simulink model "lab4_G_coeff_model_for_estimation_2019b"  (R2019b)
settings: Solver=FixedStepAuto  StartTime=0.0  StopTime=60  FixedStep=0.01  RelTol=1e-3
model workspace (MAT data in the model file):
  lab4_G_coeff_model_for_estimation_spesession : sldodialogs.data.SessionData (value not decoded)
undefined symbols (not defined in the file or in its folder): G, p
settings Model: OrderedModelArguments=off  Creator=STUDENT  LastModifiedBy=dawid

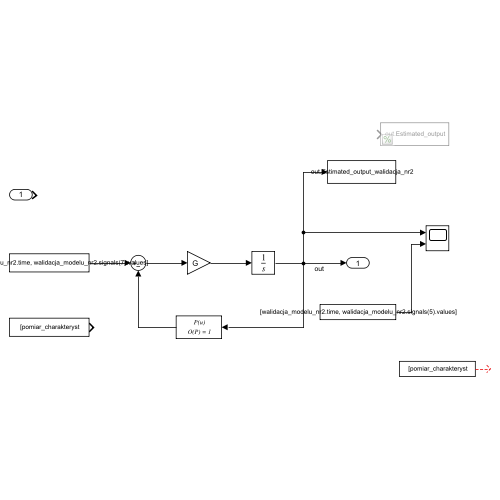
[thumbnail: Simulink's stored preview of the top-level diagram]
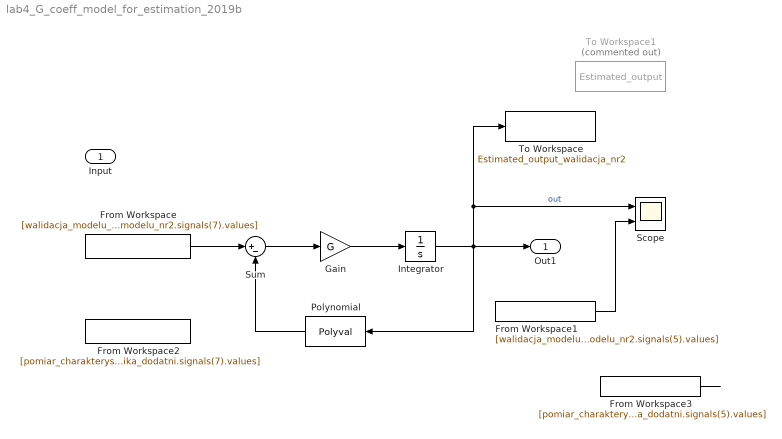
== system lab4_G_coeff_model_for_estimation_2019b ==
  Input : Inport
  From Workspace : FromWorkspace  VariableName=[walidacja_modelu_nr2.time, walidacja_modelu_nr2.signals(7).values]
  From Workspace1 : FromWorkspace  VariableName=[walidacja_modelu_nr2.time, walidacja_modelu_nr2.signals(5).values]
  From Workspace2 : FromWorkspace  VariableName=[pomiar_charakterystyki_silnika_dodatni.time, pomiar_charakterystyki_silnika_dodatni.signals(7).values]
  From Workspace3 : FromWorkspace  VariableName=[pomiar_charakterystyki_silnika_dodatni.time, pomiar_charakterystyki_silnika_dodatni.signals(5).values]
  Gain : Gain  Gain=G
  Integrator : Integrator
  Polynomial : Polyval  Coefs=p
  Scope : Scope  NumInputPorts=2
  Sum : Sum  Inputs=|+-
  To Workspace : ToWorkspace  VariableName=Estimated_output_walidacja_nr2  SaveFormat=Timeseries  SampleTime=-1
  To Workspace1 : ToWorkspace  Commented=on  VariableName=Estimated_output  SaveFormat=Timeseries  SampleTime=-1
  Out1 : Outport
  wires:
  Sum/1 -> Gain/1
  Gain/1 -> Integrator/1
  Integrator/1 -> To Workspace/1, Scope/1, Polynomial/1, Out1/1  "out"
  Polynomial/1 -> Sum/2
  From Workspace1/1 -> Scope/2
  From Workspace/1 -> Sum/1
  From Workspace3/1 -> ?
